simulink model "PcontrolModel"  (R2021b)
settings: Solver=VariableStepAuto  StartTime=0.0  StopTime=50  RelTol=1e-3
model workspace (MAT data in the model file):
  MIN = Simulink.Parameter
  MIN.DataType = 'auto'
  MIN.Complexity = 'real'
  MIN.Dimensions = [0 0]
  U = 8.05
values from neighbouring files (symbols this model uses):
  B = 0.15    [run_simulation.m]
  goal_x = 1    [run_simulation.m]
  goal_y = 1    [run_simulation.m]
  J = 0.0024    [run_simulation.m]
  Ke = 0.4870    (= 0.487)    [run_simulation.m]
  Km = Ke    (= 0.487)    [run_simulation.m]
  kr = 200    [run_simulation.m]
  ks = 200    [run_simulation.m]
  L = 0.0047    [run_simulation.m]
  r = 0.025    [run_simulation.m]
  R = 8.8696    [run_simulation.m]
  Umax = 8.05    [run_simulation.m]
  Umin = -8.05    [run_simulation.m]
settings Model: SimulationMode=accelerator  Creator=huynh  LastModifiedBy=romas

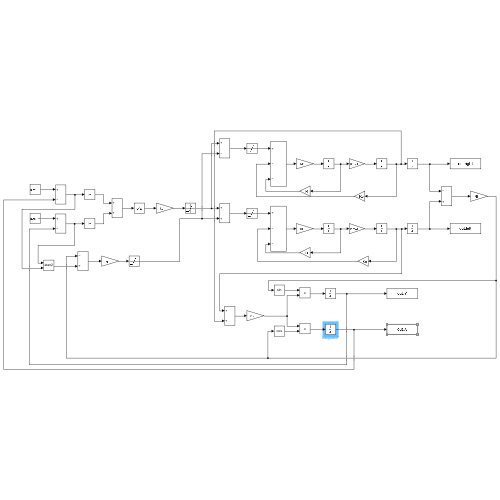
[thumbnail: Simulink's stored preview of the top-level diagram]
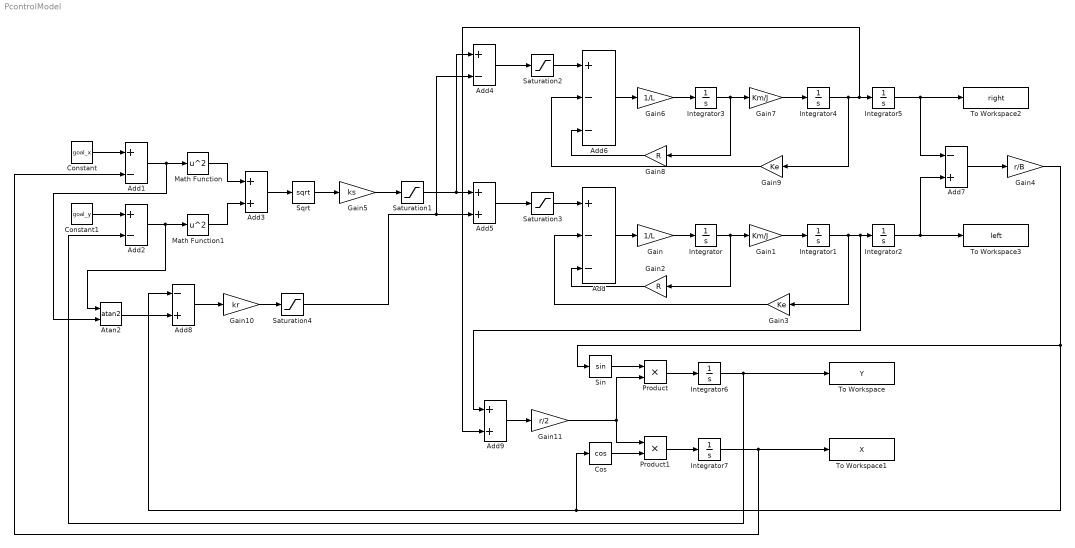
== system PcontrolModel ==
  Add : Sum  Inputs=+--
  Add1 : Sum  Inputs=+-
  Add2 : Sum  Inputs=+-
  Add3 : Sum
  Add4 : Sum  Inputs=+-
  Add5 : Sum
  Add6 : Sum  Inputs=+--
  Add7 : Sum  Inputs=-+
  Add8 : Sum  Inputs=-+
  Add9 : Sum
  Atan2 : Trigonometry  Operator=atan2
  Constant : Constant  Value=goal_x
  Constant1 : Constant  Value=goal_y
  Cos : Trigonometry  Operator=cos
  Gain : Gain  Gain=1/L
  Gain1 : Gain  Gain=Km/J
  Gain10 : Gain  Gain=kr
  Gain11 : Gain  Gain=r/2
  Gain2 : Gain  Gain=R
  Gain3 : Gain  Gain=Ke
  Gain4 : Gain  Gain=r/B
  Gain5 : Gain  Gain=ks
  Gain6 : Gain  Gain=1/L
  Gain7 : Gain  Gain=Km/J
  Gain8 : Gain  Gain=R
  Gain9 : Gain  Gain=Ke
  Integrator{,2..3,5..7} (6 alike) : Integrator
  Integrator1 : Integrator  InitialCondition=10
  Integrator4 : Integrator  InitialCondition=10
  Math Function : Math  Operator=square  SaturateOnIntegerOverflow=on
  Math Function1 : Math  Operator=square  SaturateOnIntegerOverflow=on
  Product : Product
  Product1 : Product
  Saturation1 : Saturate  UpperLimit=Umax*0.6  LowerLimit=Umin*0.6
  Saturation2 : Saturate  UpperLimit=Umax  LowerLimit=Umin
  Saturation3 : Saturate  UpperLimit=Umax  LowerLimit=Umin
  Saturation4 : Saturate  UpperLimit=Umax*0.4  LowerLimit=Umin*0.4
  Sin : Trigonometry
  Sqrt : Sqrt  SaturateOnIntegerOverflow=on
  To Workspace : ToWorkspace  VariableName=Y  SaveFormat=Timeseries  SampleTime=-1
  To Workspace1 : ToWorkspace  VariableName=X  SaveFormat=Timeseries  SampleTime=-1
  To Workspace2 : ToWorkspace  VariableName=right  SaveFormat=Timeseries  SampleTime=-1
  To Workspace3 : ToWorkspace  VariableName=left  SaveFormat=Timeseries  SampleTime=-1
  wires:
  Gain/1 -> Integrator/1
  Add/1 -> Gain/1
  Gain1/1 -> Integrator1/1
  Integrator1/1 -> Add9/1, Integrator2/1, Gain3/1
  Integrator/1 -> Gain2/1, Gain1/1
  Gain2/1 -> Add/3
  Gain3/1 -> Add/2
  Constant/1 -> Add1/1
  Constant1/1 -> Add2/1
  Add3/1 -> Sqrt/1
  Math Function/1 -> Add3/1
  Add2/1 -> Atan2/1, Math Function1/1
  Math Function1/1 -> Add3/2
  Sqrt/1 -> Gain5/1
  Gain5/1 -> Saturation1/1
  Saturation1/1 -> Add4/1, Add5/1
  Add4/1 -> Saturation2/1
  Add5/1 -> Saturation3/1
  Saturation3/1 -> Add/1
  Saturation2/1 -> Add6/1
  Integrator3/1 -> Gain8/1, Gain7/1
  Gain7/1 -> Integrator4/1
  Integrator4/1 -> Add9/2, Integrator5/1, Gain9/1
  Gain8/1 -> Add6/3
  Gain9/1 -> Add6/2
  Gain6/1 -> Integrator3/1
  Add6/1 -> Gain6/1
  Integrator5/1 -> Add7/1, To Workspace2/1
  Integrator2/1 -> To Workspace3/1, Add7/2
  Add1/1 -> Atan2/2, Math Function/1
  Atan2/1 -> Add8/2
  Add8/1 -> Gain10/1
  Gain10/1 -> Saturation4/1
  Saturation4/1 -> Add4/2, Add5/2
  Add9/1 -> Gain11/1
  Gain11/1 -> Product/2, Product1/1
  Gain4/1 -> Sin/1, Cos/1, Add8/1
  Sin/1 -> Product/1
  Cos/1 -> Product1/2
  Product/1 -> Integrator6/1
  Product1/1 -> Integrator7/1
  Integrator6/1 -> To Workspace/1, Add2/2
  Integrator7/1 -> To Workspace1/1, Add1/2
  Add7/1 -> Gain4/1
